simulink model "ServerDist2_Model"  (R2025a)
settings: Solver=VariableStepAuto  StartTime=0.0  StopTime=10.0  RelTol=1e-3
libraries: NSA_DEVS_LOGISTICS x3, NSA_DEVS_SINKS x3, NSA_DEVS_SOURCES x1
settings Model: Creator=peter  LastModifiedBy=peter

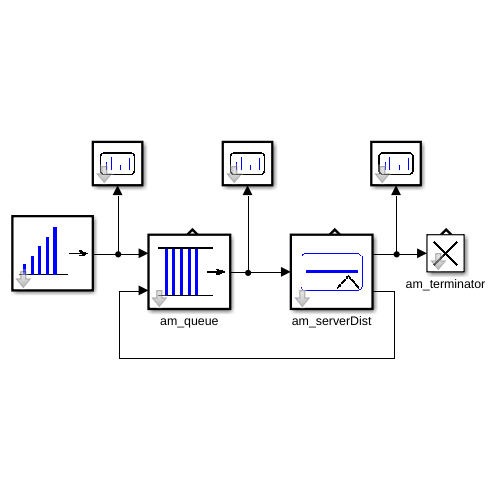
[thumbnail: Simulink's stored preview of the top-level diagram]
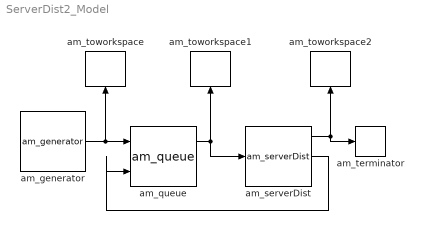
== system ServerDist2_Model ==
  am_generator : NSA_DEVS_SOURCES/am_generator  tG=0  n0=1  nG=5  tD=[0,4]  debug=0
      settings: SourceProductName=Sources
  am_queue : NSA_DEVS_LOGISTICS/am_queue  tD=[0,2]  tau=[0,1]  debug=0
      settings: SourceProductName=Logistics
  am_serverDist : NSA_DEVS_LOGISTICS/am_serverDist  distName="\"Triangular\""  distPara=[0.8,1.0,1.2]  tau=[0,1]  debug=0
      settings: SourceProductName=Logistics
  am_terminator : NSA_DEVS_LOGISTICS/am_terminator  tau=[0,1]  debug=0
      settings: SourceProductName=Logistics
  am_toworkspace : NSA_DEVS_SINKS/am_toworkspace  varname="\"gen\""  t0=0  format="\"vector\""  tau=[0,0.5]  debug=0
      settings: SourceProductName=Sinks
  am_toworkspace1 : NSA_DEVS_SINKS/am_toworkspace  varname="\"que\""  t0=0  format="\"vector\""  tau=[0,0.5]  debug=0
      settings: SourceProductName=Sinks
  am_toworkspace2 : NSA_DEVS_SINKS/am_toworkspace  varname="\"srv\""  t0=0  format="\"vector\""  tau=[0,0.5]  debug=0
      settings: SourceProductName=Sinks
  wires:
  am_queue/1 -> am_serverDist/1, am_toworkspace1/1
  am_serverDist/1 -> am_toworkspace2/1, am_terminator/1
  am_generator/1 -> am_queue/1, am_toworkspace/1
  am_serverDist/2 -> am_queue/2
